simulink model "mExportedFcnBasicNeg"  (R2013b)
settings: Solver=FixedStepDiscrete  StartTime=0.0  StopTime=0.025  FixedStep=0.001  MaxStep=.0001  RelTol=1e-3
libraries: simulink x1
Description:
  | Exporting Function-Call Subsystems
  | 
  | This example shows how to model the explicit execution of a collection
  | of blocks using function-call subsystems.
settings Model: ExtModeAutoUpdateStatusClock=off  Creator=The MathWorks Inc.  LastModifiedBy=hungdang
settings DataIOCC: SignalLoggingSaveFormat=ModelDataLogs  SaveOutput=off  SaveTime=off
settings OptimizationCC: InlineParams=on  InlineInvariantSignals=on  PassReuseOutputArgsAs=Individual arguments  ExpressionDepthLimit=2147483647  StateBitsets=on  DataBitsets=on  ActiveStateOutputEnumStorageType=Target Integer  UseTempVars=on  ZeroExternalMemoryAtStartup=off  ZeroInternalMemoryAtStartup=off  NoFixptDivByZeroProtection=on  EfficientFloat2IntCast=on  EfficientMapNaN2IntZero=off  OptimizeModelRefInitCode=on  LifeSpan=1  BufferReusableBoundary=off
settings DebuggingCC: UnderspecifiedInitializationDetection=Simplified  SolverPrmCheckMsg=none  SigSpecEnsureSampleTimeMsg=none  FcnCallInpInsideContextMsg=EnableAllAsWarning  BusObjectLabelMismatch=none  StateNameClashWarn=warning  StrictBusMsg=ErrorOnBusTreatedAsVector
settings HardwareCC: ProdIntDivRoundTo=Zero  ProdEndianess=LittleEndian  ProdHWDeviceType=Generic->32-bit Embedded Processor  TargetIntDivRoundTo=Zero  TargetEndianess=LittleEndian  TargetHWDeviceType=Generic->32-bit Embedded Processor
settings SFSimCC: SimParseCustomCode=off
settings RTWCC: SystemTargetFile=ert.tlc  TemplateMakefile=ert_default_tmf  Description=Embedded Coder (no auto configuration)  GenerateReport=on  RTWVerbose=off  ProcessScript=ert_make_rtw_hook  IncludeHyperlinkInReport=on  LaunchReport=on  PortableWordSizes=on
settings CodeAppCC: ForceParamTrailComments=on  IgnoreCustomStorageClasses=off  IgnoreTestpoints=on  SimulinkDataObjDesc=on  CustomSymbolStrGlobalVar=rt$N$M  CustomSymbolStrType=$N$M  CustomSymbolStrFcn=$N$M$F  CustomSymbolStrMacro=$N$M  InsertBlockDesc=on  InternalIdentifier=Classic
settings ERTTargetCC: TargetFcnLib=ansi_tfl_tmw.mat  CodeReplacementLibrary=ANSI_C  UtilityFuncGeneration=Shared location  GenerateSampleERTMain=on  IncludeMdlTerminateFcn=off  SupportNonFinite=off  SupportComplex=off  InlinedParameterPlacement=NonHierarchical  ERTCustomFileTemplate=example_file_process.tlc  ERTFilePackagingFormat=CompactWithDataFile

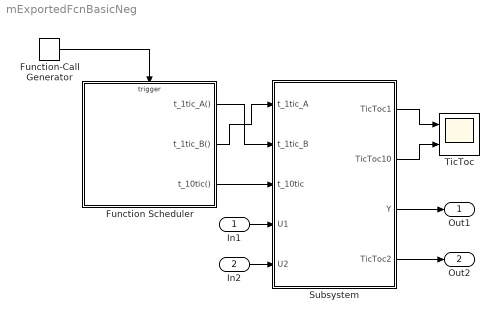
== system mExportedFcnBasicNeg ==
  In1 : Inport  OutDataTypeStr=double  PortDimensions=1  SampleTime=0.001
  In2 : Inport  Port=2  OutDataTypeStr=double  PortDimensions=1  SampleTime=0.001
  Function Scheduler : Stateflow chart  TreatAsAtomicUnit=on
  Function-Call Generator : simulink/Ports & Subsystems/Function-Call Generator  sample_time=0.001  numberOfIterations=1
  Subsystem : Subsystem
  TicToc : Scope  NumInputPorts=2
      settings: TimeRange=0.025  YMin=0~-1  YMax=1~1
  Out1 : Outport
  Out2 : Outport  Port=2
  wires:
  Function-Call Generator/1 -> Function Scheduler/Trigger
  In1/1 -> Subsystem/4(U1)
  In2/1 -> Subsystem/5(U2)
  Subsystem/3(Y) -> Out1/1
  Function Scheduler/3(t_10tic()) -> Subsystem/3(t_10tic)
  Subsystem/1(TicToc1) -> TicToc/1
  Subsystem/2(TicToc10) -> TicToc/2
  Subsystem/4(TicToc2) -> Out2/1
  Function Scheduler/1(t_1tic_A()) -> Subsystem/2(t_1tic_B)
  Function Scheduler/2(t_1tic_B()) -> Subsystem/1(t_1tic_A)

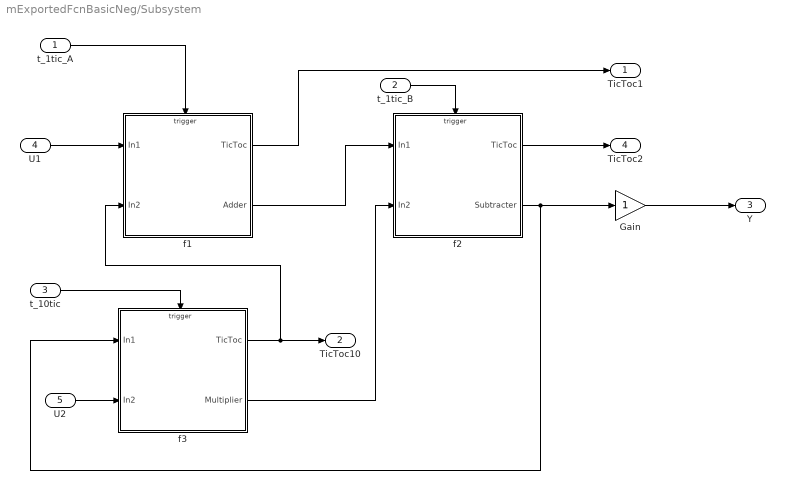
== system mExportedFcnBasicNeg/Subsystem ==
  t_1tic_A : Inport
  t_1tic_B : Inport  Port=2
  t_10tic : Inport  Port=3
  U1 : Inport  Port=4
  U2 : Inport  Port=5
  Gain : Gain
  f1 : Subsystem  TreatAsAtomicUnit=on  RTWFcnName=foo
  f2 : Subsystem  TreatAsAtomicUnit=on  RTWFcnName=foo
  f3 : Subsystem  TreatAsAtomicUnit=on  RTWFcnName=foo
  TicToc1 : Outport
  TicToc10 : Outport  Port=2
  Y : Outport  Port=3
  TicToc2 : Outport  Port=4
  wires:
  t_10tic/1 -> f3/Trigger
  U2/1 -> f3/2(In2)
  f2/2(Subtracter) -> Gain/1, f3/1(In1)
  f1/2(Adder) -> f2/1(In1)
  f3/2(Multiplier) -> f2/2(In2)
  t_1tic_A/1 -> f1/Trigger
  f3/1(TicToc) -> f1/2(In2), TicToc10/1
  f2/1(TicToc) -> TicToc2/1
  f1/1(TicToc) -> TicToc1/1
  t_1tic_B/1 -> f2/Trigger
  U1/1 -> f1/1(In1)
  Gain/1 -> Y/1

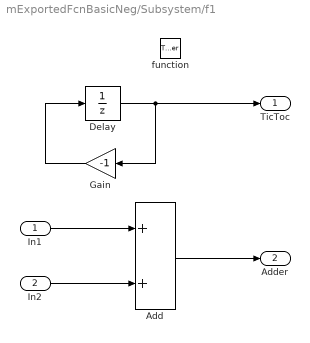
== system mExportedFcnBasicNeg/Subsystem/f1 ==
  In1 : Inport
  In2 : Inport  Port=2
  function : TriggerPort  TriggerType=function-call
  Add : Sum
  Delay : UnitDelay  InitialCondition=1  SampleTime=-1
  Gain : Gain  Gain=-1  OutDataTypeStr=fixdt(1,8,0)
  TicToc : Outport  InitialOutput=0
  Adder : Outport  Port=2  InitialOutput=0
  wires:
  Add/1 -> Adder/1
  Gain/1 -> Delay/1
  Delay/1 -> TicToc/1, Gain/1
  In1/1 -> Add/1
  In2/1 -> Add/2

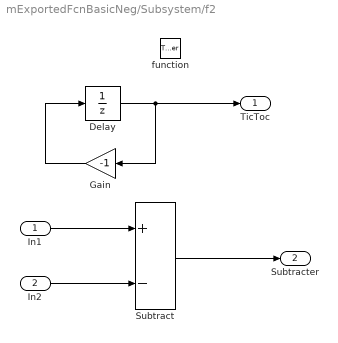
== system mExportedFcnBasicNeg/Subsystem/f2 ==
  In1 : Inport
  In2 : Inport  Port=2
  function : TriggerPort  TriggerType=function-call
  Delay : UnitDelay  InitialCondition=1  SampleTime=-1
  Gain : Gain  Gain=-1  OutDataTypeStr=fixdt(1,8,0)
  Subtract : Sum  Inputs=+-
  TicToc : Outport  InitialOutput=0
  Subtracter : Outport  Port=2  InitialOutput=0
  wires:
  In2/1 -> Subtract/2
  In1/1 -> Subtract/1
  Delay/1 -> Gain/1, TicToc/1
  Gain/1 -> Delay/1
  Subtract/1 -> Subtracter/1

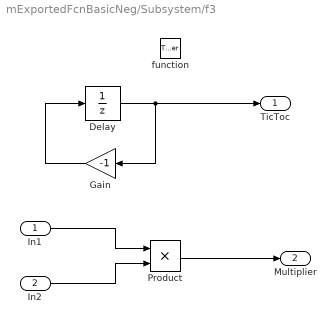
== system mExportedFcnBasicNeg/Subsystem/f3 ==
  In1 : Inport
  In2 : Inport  Port=2
  function : TriggerPort  TriggerType=function-call
  Delay : UnitDelay  InitialCondition=1  SampleTime=-1
  Gain : Gain  Gain=-1  OutDataTypeStr=fixdt(1,8,0)
  Product : Product  Inputs=**  OutDataTypeStr=Inherit: Same as first input
  TicToc : Outport  InitialOutput=0
  Multiplier : Outport  Port=2  InitialOutput=0
  wires:
  In2/1 -> Product/2
  In1/1 -> Product/1
  Delay/1 -> Gain/1, TicToc/1
  Gain/1 -> Delay/1
  Product/1 -> Multiplier/1

== stateflow chart mExportedFcnBasicNeg/Function Scheduler ==
  settings: initializeOutput=1
  state OneTic [parallel]
    entry: t_1tic_B; t_1tic_A;
    on every(1,tic):
    t_1tic_B; t_1tic_A;
    settings: executionOrder=1
  state TenTic [parallel]
    entry: t_10tic;
    on every(10,tic): t_10tic;
    settings: executionOrder=2
  events: tic input FUNCTION_CALL_EVENT; t_1tic_A output FUNCTION_CALL_EVENT; t_1tic_B output FUNCTION_CALL_EVENT; t_10tic output FUNCTION_CALL_EVENT
